simulink model "ex1c"  (R2015a)
settings: Solver=ode45  StartTime=0.0  StopTime=10.0  RelTol=1e-3
values from neighbouring files (symbols this model uses):
  D = [1 2 4]    [ex1.m]
  k = 1    [ex1.m]
  m = 1    [ex1.m]
settings Model: Creator=martinspedro  LastModifiedBy=martinspedro

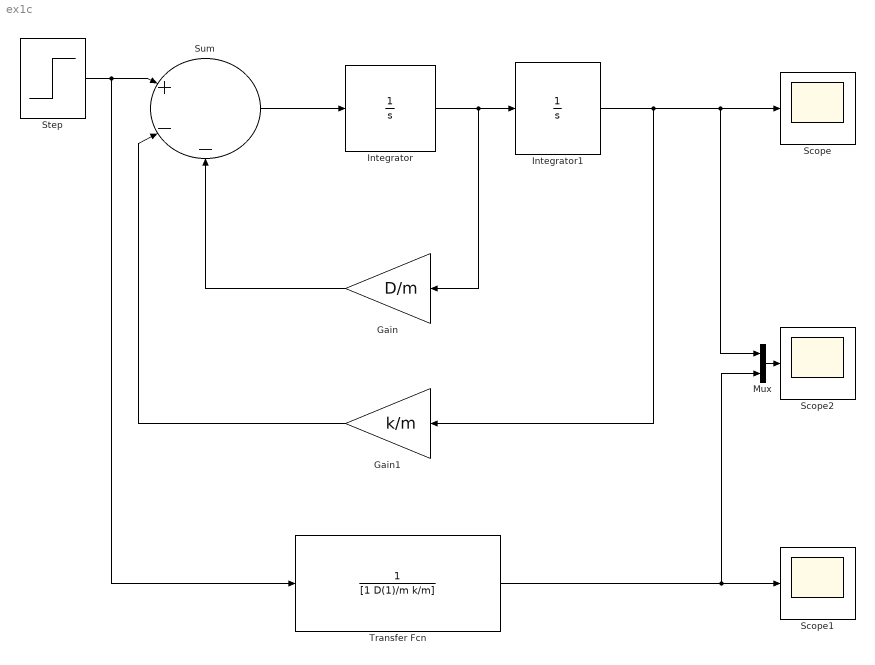
== system ex1c ==
  Gain : Gain  Gain=D/m
  Gain1 : Gain  Gain=k/m
  Integrator : Integrator
  Integrator1 : Integrator
  Mux : Mux  Inputs=2
  Scope : Scope
      settings: ShowLegends=on  ScrollMode=on
  Scope1 : Scope
      settings: ShowLegends=on
  Scope2 : Scope
      settings: ShowLegends=on  TimeRange=10  YMin=0  YMax=1.2  SaveName=ScopeData2
  Step : Step  Time=0  SampleTime=0
  Sum : Sum  Inputs=|+--
  Transfer Fcn : TransferFcn  Denominator=[1 D(1)/m k/m]
  wires:
  Sum/1 -> Integrator/1
  Integrator/1 -> Gain/1, Integrator1/1
  Gain1/1 -> Sum/2
  Gain/1 -> Sum/3
  Step/1 -> Transfer Fcn/1, Sum/1
  Transfer Fcn/1 -> Scope1/1, Mux/2
  Mux/1 -> Scope2/1
  Integrator1/1 -> Gain1/1, Mux/1, Scope/1
